simulink model "TDPBehaviourSim2"  (R2020b)
settings: Solver=FixedStepAuto  StartTime=0.0  StopTime=200  FixedStep=sampleTime  RelTol=1e-3  EnableMultiTasking=on
values from neighbouring files (symbols this model uses):
  angThresh = pi/16    (= 0.196349540849)    [GameParameters.m]
  attackerKickSpeed = 0.3    [GameParameters.m]
  AwayFormation1 = [9.5 4 pi ... (first row only)    [FormationPoses.m]    (also in GameParameters.m)
  ballAngleNoise = pi/24    (= 0.1308996939)    [GameParameters.m]
  ballThresh = playerRadius + 0.03    (= 0.11)    [GameParameters.m]
  ballVelNoise = 0.05    [GameParameters.m]
  distThresh = 0.1    [GameParameters.m]
  fieldCenter = [mean(fieldLimitsX) mean(fieldLimitsY)]    [GameParameters.m]
  fieldLimitsX = [1 10]    [GameParameters.m]
  fieldLimitsY = [1 7]    [GameParameters.m]
  goalPosts = [1  2.7 2 ... (first row only)    [GameParameters.m]
  HomeFormation1 = [1.5 4 0 ... (first row only)    [FormationPoses.m]    (also in GameParameters.m)
  maxSpeed = 0.1    [GameParameters.m]
  maxTurnSpeed = 0.05    [GameParameters.m]
  playerIdx = (0:8)    [GameParameters.m]
  playerRadius = 0.08    [GameParameters.m]
  sampleTime = 0.1    [GameParameters.m]
undefined symbols (not defined in the file or in its folder): DiscIntNeverNeededParam
libraries: mobileRoboticsLib x33, soccerRobotLib x16
(part 1 of 2)
settings Model: SimulationMode=accelerator  SnapshotBufferSize=20  Creator=2683935i  LastModifiedBy=2683935i
settings SolverCC: AutoInsertRateTranBlk=on
settings DataIOCC: SaveOutput=off  SaveTime=off
settings OptimizationCC: DefaultParameterBehavior=Inlined  InlineInvariantSignals=on  EnhancedBackFolding=on  PassReuseOutputArgsAs=Individual arguments  StateBitsets=on  DataBitsets=on  ZeroExternalMemoryAtStartup=off  ZeroInternalMemoryAtStartup=off  NoFixptDivByZeroProtection=on  LifeSpan=1  OptimizeBlockOrder=speed  DifferentSizesBufferReuse=on  EfficientTunableParamExpr=on
settings DebuggingCC: ParameterTunabilityLossMsg=error  UnderSpecifiedDimensionMsg=warning
settings HardwareCC: ProdBitPerPointer=32  ProdBitPerSizeT=32  ProdBitPerPtrDiffT=32  ProdLargestAtomicFloat=None  ProdIntDivRoundTo=Floor  ProdWordSize=32  ProdHWDeviceType=Generic->Custom
settings SFSimCC: MATLABDynamicMemAlloc=off
settings RTWCC: Description=Embedded Coder  SystemTargetFile=ert.tlc  TLCOptions=-p0  GenCodeOnly=on  TemplateMakefile=ert_default_tmf  GenerateReport=on  RTWVerbose=off  IncludeHyperlinkInReport=on  LaunchReport=on
settings CodeAppCC: ForceParamTrailComments=on  IgnoreCustomStorageClasses=off  OperatorAnnotations=on  SimulinkDataObjDesc=on  SFDataObjDesc=on  CustomSymbolStrGlobalVar=rt$N$M  CustomSymbolStrType=$N$M  CustomSymbolStrFcn=$N$M$F  CustomSymbolStrMacro=$N$M  InsertBlockDesc=on
settings ERTTargetCC: TargetLangStandard=C99 (ISO)  GenerateSampleERTMain=on  IncludeMdlTerminateFcn=off  SuppressErrorStatus=on  SupportAbsoluteTime=off  PurelyIntegerCode=on  SupportNonFinite=off  SupportComplex=off  InlinedParameterPlacement=NonHierarchical  RootIOFormat=Structure reference  ERTCustomFileTemplate=example_file_process.tlc

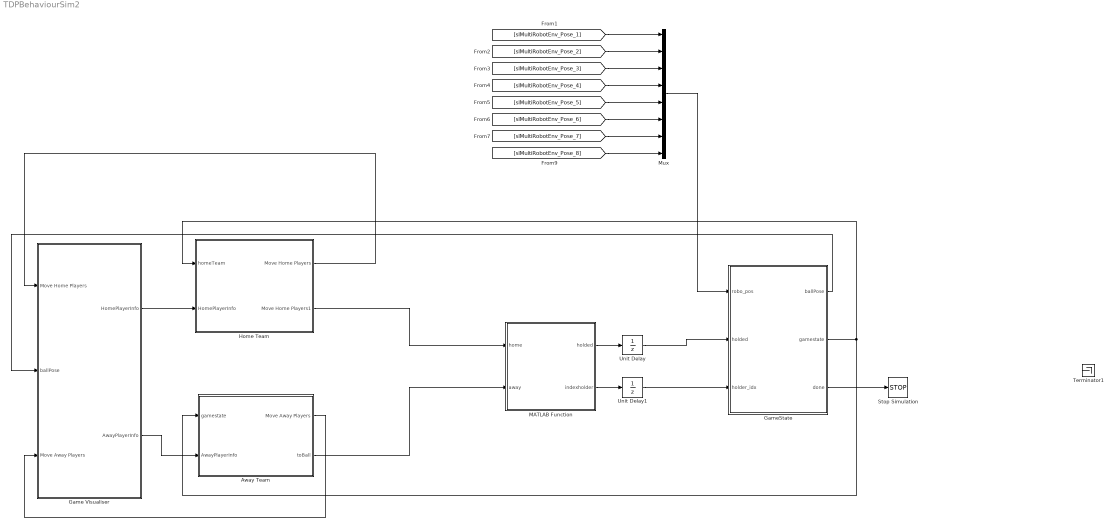
== system TDPBehaviourSim2 ==
  Away Team : Subsystem
  Game Visualiser : Subsystem
  GameState : Stateflow chart  TreatAsAtomicUnit=on
  Home Team : Subsystem
  MATLAB Function : MATLAB Function  TreatAsAtomicUnit=on
  Mux : Mux  Inputs=8
  Stop Simulation : Stop
  Terminator1 : Terminator
  Unit Delay : UnitDelay  SampleTime=-1  HasFrameUpgradeWarning=on
  Unit Delay1 : UnitDelay  SampleTime=-1  HasFrameUpgradeWarning=on
  wires:
  Home Team/1(Move Home Players) -> Game Visualiser/1(Move Home Players)
  Game Visualiser/1(HomePlayerInfo) -> Home Team/2(HomePlayerInfo)
  Game Visualiser/2(AwayPlayerInfo) -> Away Team/2(AwayPlayerInfo)
  [slMultiRobotEnv_Pose_4] -> Mux/4
  [slMultiRobotEnv_Pose_8] -> Mux/8
  [slMultiRobotEnv_Pose_1] -> Mux/1
  Mux/1 -> GameState/1(robo_pos)
  [slMultiRobotEnv_Pose_2] -> Mux/2
  [slMultiRobotEnv_Pose_3] -> Mux/3
  GameState/1(ballPose) -> Game Visualiser/2(ballPose)
  Home Team/2(Move Home Players1) -> MATLAB Function/1(home)
  GameState/3(done) -> Stop Simulation/1
  [slMultiRobotEnv_Pose_5] -> Mux/5
  [slMultiRobotEnv_Pose_6] -> Mux/6
  [slMultiRobotEnv_Pose_7] -> Mux/7
  GameState/2(gamestate) -> Away Team/1(gamestate), Home Team/1(homeTeam)
  MATLAB Function/2(indexholder) -> Unit Delay1/1
  Unit Delay1/1 -> GameState/3(holder_idx)
  MATLAB Function/1(holded) -> Unit Delay/1
  Unit Delay/1 -> GameState/2(holded)
  Away Team/2(toBall) -> MATLAB Function/2(away)
  Away Team/1(Move Away Players) -> Game Visualiser/3(Move Away Players)

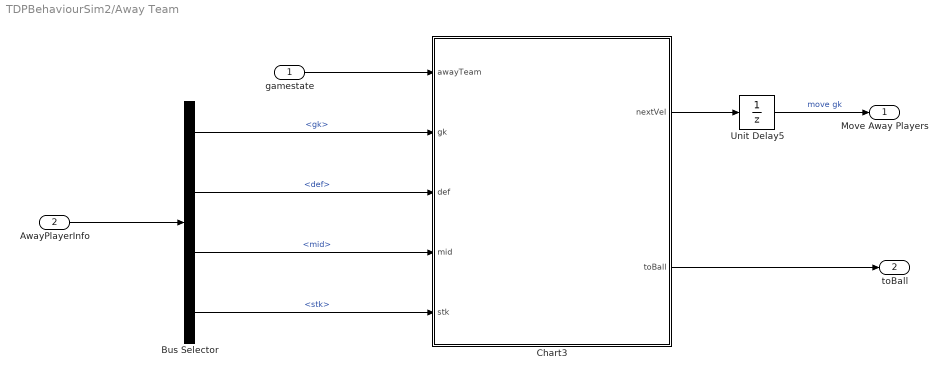
== system TDPBehaviourSim2/Away Team ==
  gamestate : Inport
  AwayPlayerInfo : Inport  Port=2
  Bus Selector : BusSelector  OutputSignals=gk,def,mid,stk
  Chart3 : Stateflow chart  TreatAsAtomicUnit=on
      settings: PortSchema="{\"entries\":[{\"content\":{\"sides\":[{\"content\":{\"connectorIds\":[\"In1\",\"In2\",\"In3\",\"In4\",\"In5\"]},\"type\":\"ConnectorPlacement.EquallySpacedRectSide\",\"uuid\":\"ebe0e1cb-6371-4bd3-ace0-cc5b71048631\"},{\"content\":{\"connectorIds\":[\"Out2\",\"Out1\"],\"side\":\"RIGHT\"},\"type\":\"ConnectorPlacement.EquallySpacedRectSide\",\"uuid\":\"57a2731b-5a64-47ed-8ccc-f0829cfb4352\"},{\"content\":{\"connectorIds\":[],\"side\":\"TOP\"},\"type\":\"ConnectorPlacement.EquallySpacedRectSide\",\"uuid\":\"36798d0f-f2da-4938-9b0d-f712c5a2717d\"},{\"content\":{\"connectorIds\":[],\"side\":\"HIDDEN\"},\"type\":\"ConnectorPlacement.EquallySpacedRectSide\",\"uuid\":\"e7d6e691-e5a0-4113-9f42-d5d110a4eaa7\"}]},\"type\":\"ConnectorPlacement.EquallySpacedConnector\",\"uuid\":\"d2e32adf-2fdb-404f-9614-4542aac92af5\"}],\"packageUris\":[\"http://schema.mathworks.com/mf0/Connector/R2020b\"],\"version\":\"1.0\"}"
  Unit Delay5 : UnitDelay  SampleTime=-1  HasFrameUpgradeWarning=on
  Move Away Players : Outport
  toBall : Outport  Port=2
  wires:
  Chart3/2(nextVel) -> Unit Delay5/1
  Unit Delay5/1 -> Move Away Players/1  "move gk"
  gamestate/1 -> Chart3/1(awayTeam)
  AwayPlayerInfo/1 -> Bus Selector/1
  Chart3/1(toBall) -> toBall/1
  Bus Selector/1 -> Chart3/2(gk)  "<gk>"
  Bus Selector/2 -> Chart3/3(def)  "<def>"
  Bus Selector/3 -> Chart3/4(mid)  "<mid>"
  Bus Selector/4 -> Chart3/5(stk)  "<stk>"

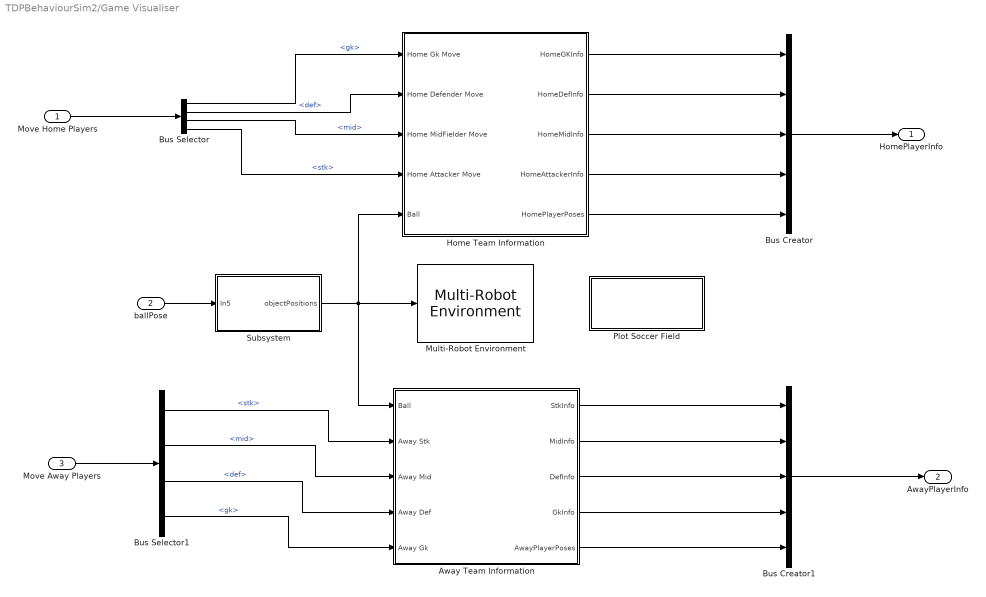
== system TDPBehaviourSim2/Game Visualiser ==
  Move Home Players : Inport
  ballPose : Inport  Port=2
  Move Away Players : Inport  Port=3
  Away Team Information : Subsystem
  Bus Creator : BusCreator  Inputs=5
  Bus Creator1 : BusCreator  Inputs=5
  Bus Selector : BusSelector  OutputSignals=gk,def,mid,stk
  Bus Selector1 : BusSelector  OutputSignals=stk,mid,def,gk
  Home Team Information : Subsystem
  Multi-Robot Environment : mobileRoboticsLib/Environments/Multi-Robot Environment  numRobots=numPlayers  mapName=map  showWaypoints=off  showObjects=on  objectColors=objColors  objectMarkers='o^^^^'  showRobotIds=on  plotSensorLines=off
      settings: SourceProductName=Mobile Robotics Simulation Toolbox
  Plot Soccer Field : MATLAB Function  TreatAsAtomicUnit=on
  Subsystem : Subsystem
  HomePlayerInfo : Outport
  AwayPlayerInfo : Outport  Port=2
  wires:
  Home Team Information/1(HomeGKInfo) -> Bus Creator/1
  Home Team Information/2(HomeDefInfo) -> Bus Creator/2
  Home Team Information/3(HomeMidInfo) -> Bus Creator/3
  Home Team Information/4(HomeAttackerInfo) -> Bus Creator/4
  Home Team Information/5(HomePlayerPoses) -> Bus Creator/5
  Away Team Information/1(StkInfo) -> Bus Creator1/1
  Away Team Information/2(MidInfo) -> Bus Creator1/2
  Away Team Information/3(DefInfo) -> Bus Creator1/3
  Away Team Information/4(GkInfo) -> Bus Creator1/4
  Away Team Information/5(AwayPlayerPoses) -> Bus Creator1/5
  Subsystem/1(objectPositions) -> Multi-Robot Environment/1, Away Team Information/1(Ball), Home Team Information/5(Ball)
  ballPose/1 -> Subsystem/1(In5)
  Move Away Players/1 -> Bus Selector1/1
  Bus Creator/1 -> HomePlayerInfo/1
  Bus Creator1/1 -> AwayPlayerInfo/1
  Move Home Players/1 -> Bus Selector/1
  Bus Selector/1 -> Home Team Information/1(Home Gk Move)  "<gk>"
  Bus Selector/2 -> Home Team Information/2(Home Defender Move)  "<def>"
  Bus Selector/3 -> Home Team Information/3(Home MidFielder Move)  "<mid>"
  Bus Selector/4 -> Home Team Information/4(Home Attacker Move)  "<stk>"
  Bus Selector1/1 -> Away Team Information/2(Away Stk)  "<stk>"
  Bus Selector1/2 -> Away Team Information/3(Away Mid)  "<mid>"
  Bus Selector1/3 -> Away Team Information/4(Away Def)  "<def>"
  Bus Selector1/4 -> Away Team Information/5("Away Gk ")  "<gk>"

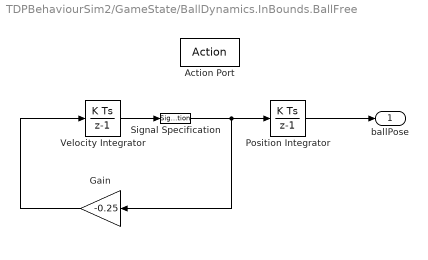
== system TDPBehaviourSim2/GameState/BallDynamics.InBounds.BallFree ==
  Action Port : ActionPort
      settings: CopyFcn=Stateflow.SLINSF.SimulinkMan.removeBlockPreDeleteFcn  PreDeleteFcn=Stateflow.SLINSF.SimulinkMan.unsafePredeleteFcn
  Gain : Gain  Gain=-0.25
  Position Integrator : DiscreteIntegrator  InitialCondition=fieldCenter  SampleTime=-1  StateName=ballPos  ICPrevOutput=DiscIntNeverNeededParam  ICPrevScaledInput=DiscIntNeverNeededParam
  Signal Specification : SignalSpecification  Dimensions=[1 2]
  Velocity Integrator : DiscreteIntegrator  InitialCondition=[0 0]  SampleTime=-1  StateName=ballVel  ICPrevOutput=DiscIntNeverNeededParam  ICPrevScaledInput=DiscIntNeverNeededParam
  ballPose : Outport  VectorParamsAs1DForOutWhenUnconnected=off
  wires:
  Gain/1 -> Velocity Integrator/1
  Velocity Integrator/1 -> Signal Specification/1
  Position Integrator/1 -> ballPose/1
  Signal Specification/1 -> Position Integrator/1, Gain/1

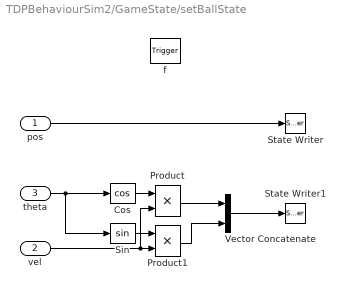
== system TDPBehaviourSim2/GameState/setBallState ==
  pos : Inport  OutDataTypeStr=double  PortDimensions=[1 2]
  vel : Inport  Port=2  OutDataTypeStr=double  PortDimensions=1
  theta : Inport  Port=3  OutDataTypeStr=double  PortDimensions=1
  f : TriggerPort  TriggerType=function-call  VariantControl=(inherit)
      settings: CopyFcn=Stateflow.SLINSF.SimulinkMan.removeBlockPreDeleteFcn  PreDeleteFcn=Stateflow.SLINSF.SimulinkMan.unsafePredeleteFcn
  Cos : Trigonometry  Operator=cos
  Product : Product
  Product1 : Product
  Sin : Trigonometry
  State Writer : StateWriter  StateOwnerBlock=../../BallDynamics.InBounds.BallFree/Position Integrator  StateName=ballPos
  State Writer1 : StateWriter  StateOwnerBlock=../../BallDynamics.InBounds.BallFree/Velocity Integrator  StateName=ballVel
  Vector Concatenate : Concatenate  Mode=Multidimensional array  ConcatenateDimension=2
  wires:
  Vector Concatenate/1 -> State Writer1/1
  Product1/1 -> Vector Concatenate/2
  Product/1 -> Vector Concatenate/1
  theta/1 -> Cos/1, Sin/1
  Sin/1 -> Product1/1
  vel/1 -> Product1/2, Product/2
  Cos/1 -> Product/1
  pos/1 -> State Writer/1

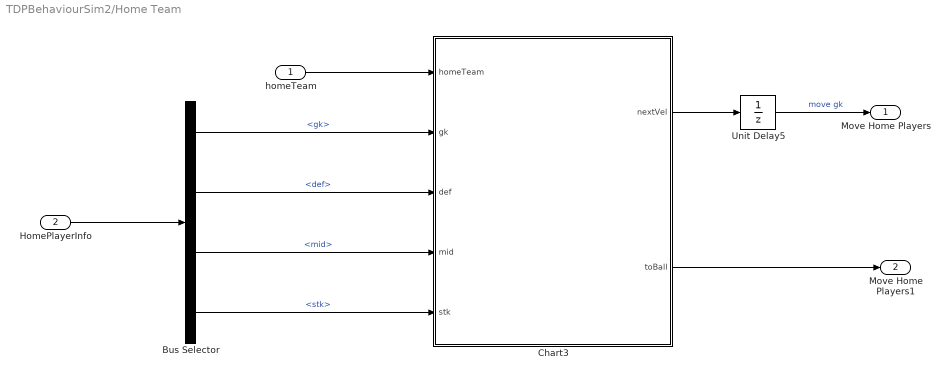
== system TDPBehaviourSim2/Home Team ==
  homeTeam : Inport
  HomePlayerInfo : Inport  Port=2
  Bus Selector : BusSelector  OutputSignals=gk,def,mid,stk
  Chart3 : Stateflow chart  TreatAsAtomicUnit=on
      settings: PortSchema="{\"entries\":[{\"content\":{\"sides\":[{\"content\":{\"connectorIds\":[\"In1\",\"In2\",\"In3\",\"In4\",\"In5\"]},\"type\":\"ConnectorPlacement.EquallySpacedRectSide\",\"uuid\":\"ebe0e1cb-6371-4bd3-ace0-cc5b71048631\"},{\"content\":{\"connectorIds\":[\"Out2\",\"Out1\"],\"side\":\"RIGHT\"},\"type\":\"ConnectorPlacement.EquallySpacedRectSide\",\"uuid\":\"57a2731b-5a64-47ed-8ccc-f0829cfb4352\"},{\"content\":{\"connectorIds\":[],\"side\":\"TOP\"},\"type\":\"ConnectorPlacement.EquallySpacedRectSide\",\"uuid\":\"36798d0f-f2da-4938-9b0d-f712c5a2717d\"},{\"content\":{\"connectorIds\":[],\"side\":\"HIDDEN\"},\"type\":\"ConnectorPlacement.EquallySpacedRectSide\",\"uuid\":\"e7d6e691-e5a0-4113-9f42-d5d110a4eaa7\"}]},\"type\":\"ConnectorPlacement.EquallySpacedConnector\",\"uuid\":\"d2e32adf-2fdb-404f-9614-4542aac92af5\"}],\"packageUris\":[\"http://schema.mathworks.com/mf0/Connector/R2020b\"],\"version\":\"1.0\"}"
  Unit Delay5 : UnitDelay  SampleTime=-1  HasFrameUpgradeWarning=on
  Move Home Players : Outport
  Move Home Players1 : Outport  Port=2
  wires:
  HomePlayerInfo/1 -> Bus Selector/1
  Bus Selector/2 -> Chart3/3(def)  "<def>"
  Bus Selector/3 -> Chart3/4(mid)  "<mid>"
  Bus Selector/4 -> Chart3/5(stk)  "<stk>"
  Bus Selector/1 -> Chart3/2(gk)  "<gk>"
  Chart3/1(toBall) -> Move Home Players1/1
  Chart3/2(nextVel) -> Unit Delay5/1
  Unit Delay5/1 -> Move Home Players/1  "move gk"
  homeTeam/1 -> Chart3/1(homeTeam)

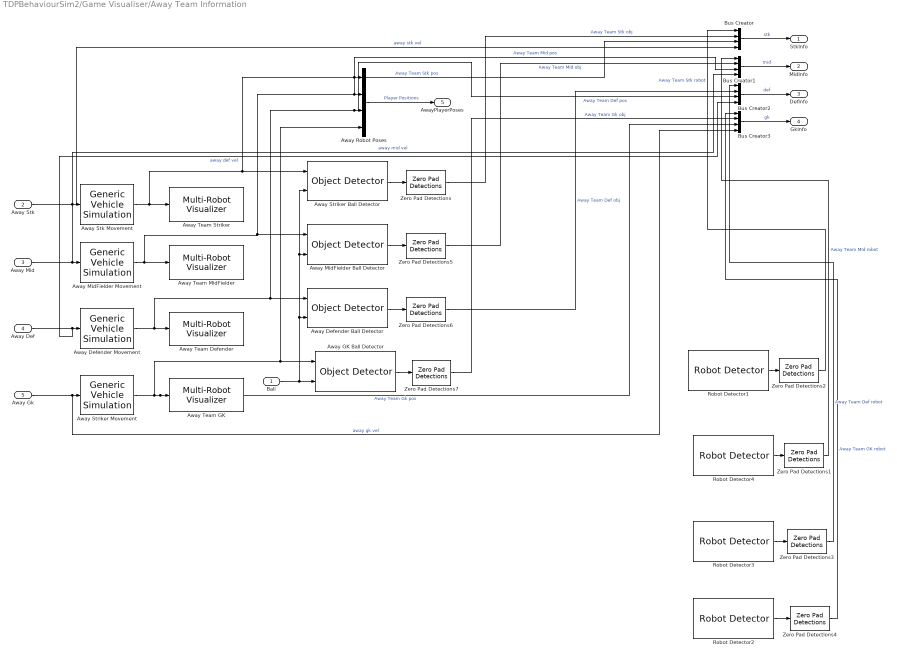
== system TDPBehaviourSim2/Game Visualiser/Away Team Information ==
  Ball : Inport
  Away Stk : Inport  Port=2
  Away Mid : Inport  Port=3
  Away Def : Inport  Port=4
  "Away Gk " : Inport  Port=5
  Away Defender Ball Detector : mobileRoboticsLib/Environments/Object Detector  mapName=map  sensorOffset=objDetectorOffset  sensorAngle=objDetectorAngle  fieldOfView=objDetectorFOV  maxRange=objDetectorRange  maxDetections=objDetectorMaxHits  sampleTime=sampleTime
      settings: SourceProductName=Mobile Robotics Simulation Toolbox
  Away Defender Movement : mobileRoboticsLib/Utilities/Generic Vehicle Simulation  initX=AwayFormation1(2,1)  initY=AwayFormation1(2,2)  initAngle=AwayFormation1(2,3)  Ts=sampleTime
      settings: SourceProductName=Mobile Robotics Simulation Toolbox
  Away GK Ball Detector : mobileRoboticsLib/Environments/Object Detector  mapName=map  sensorOffset=objDetectorOffset  sensorAngle=objDetectorAngle  fieldOfView=objDetectorFOV  maxRange=objDetectorRange  maxDetections=objDetectorMaxHits  sampleTime=sampleTime
      settings: SourceProductName=Mobile Robotics Simulation Toolbox
  Away MidFielder Ball Detector : mobileRoboticsLib/Environments/Object Detector  mapName=map  sensorOffset=objDetectorOffset  sensorAngle=objDetectorAngle  fieldOfView=objDetectorFOV  maxRange=objDetectorRange  maxDetections=objDetectorMaxHits  sampleTime=sampleTime
      settings: SourceProductName=Mobile Robotics Simulation Toolbox
  Away MidFielder Movement : mobileRoboticsLib/Utilities/Generic Vehicle Simulation  initX=AwayFormation1(3,1)  initY=AwayFormation1(3,2)  initAngle=AwayFormation1(3,3)  Ts=sampleTime
      settings: SourceProductName=Mobile Robotics Simulation Toolbox
  Away Robot Poses : BusCreator  Inputs=4
  Away Stk Movement : mobileRoboticsLib/Utilities/Generic Vehicle Simulation  initX=AwayFormation1(4,1)  initY=AwayFormation1(4,2)  initAngle=AwayFormation1(4,3)  Ts=sampleTime
      settings: SourceProductName=Mobile Robotics Simulation Toolbox
  Away Striker Ball Detector : mobileRoboticsLib/Environments/Object Detector  mapName=map  sensorOffset=objDetectorOffset  sensorAngle=objDetectorAngle  fieldOfView=objDetectorFOV  maxRange=objDetectorRange  maxDetections=objDetectorMaxHits  sampleTime=sampleTime
      settings: SourceProductName=Mobile Robotics Simulation Toolbox
  Away Striker Movement : mobileRoboticsLib/Utilities/Generic Vehicle Simulation  initX=AwayFormation1(1,1)  initY=AwayFormation1(1,2)  initAngle=AwayFormation1(1,3)  Ts=sampleTime
      settings: SourceProductName=Mobile Robotics Simulation Toolbox
  Away Team Defender : mobileRoboticsLib/Environments/Multi-Robot Visualizer  idx=7  radius=playerRadius  robotColor=awayTeamColor  showTraj=on  hasLidar=off  sensorOffset=[0,0]  scanAngles=[-pi/4 0 pi/4]  maxNumScans=0  hasObjDetector=on  objDetectorOffset=objDetectorOffset  objDetectorAngle=objDetectorAngle  objDetectorFOV=objDetectorFOV  objDetectorMaxRange=objDetectorRange  hasRobotDetector=on  robotDetectorOffset=robotDetectorOffset  robotDetectorAngle=robotDetectorAngle  robotDetectorFOV=robotDetectorFOV  robotDetectorMaxRange=robotDetectorMaxHits  robotDetectorNumDetections=0
      settings: SourceProductName=Mobile Robotics Simulation Toolbox
  Away Team GK : mobileRoboticsLib/Environments/Multi-Robot Visualizer  idx=8  radius=playerRadius  robotColor=awayGKColor  showTraj=on  hasLidar=off  sensorOffset=[0,0]  scanAngles=[-pi/4 0 pi/4]  maxNumScans=0  hasObjDetector=on  objDetectorOffset=objDetectorOffset  objDetectorAngle=objDetectorAngle  objDetectorFOV=objDetectorFOV  objDetectorMaxRange=objDetectorRange  hasRobotDetector=on  robotDetectorOffset=robotDetectorOffset  robotDetectorAngle=robotDetectorAngle  robotDetectorFOV=robotDetectorFOV  robotDetectorMaxRange=robotDetectorMaxHits  robotDetectorNumDetections=0
      settings: SourceProductName=Mobile Robotics Simulation Toolbox
  Away Team MidFielder : mobileRoboticsLib/Environments/Multi-Robot Visualizer  idx=6  radius=playerRadius  robotColor=awayTeamColor  showTraj=on  hasLidar=off  sensorOffset=[0,0]  scanAngles=[-pi/4 0 pi/4]  maxNumScans=0  hasObjDetector=on  objDetectorOffset=objDetectorOffset  objDetectorAngle=objDetectorAngle  objDetectorFOV=objDetectorFOV  objDetectorMaxRange=objDetectorRange  hasRobotDetector=on  robotDetectorOffset=robotDetectorOffset  robotDetectorAngle=robotDetectorAngle  robotDetectorFOV=robotDetectorFOV  robotDetectorMaxRange=robotDetectorMaxHits  robotDetectorNumDetections=0
      settings: SourceProductName=Mobile Robotics Simulation Toolbox
  Away Team Striker : mobileRoboticsLib/Environments/Multi-Robot Visualizer  idx=5  radius=playerRadius  robotColor=awayTeamColor  showTraj=on  hasLidar=off  sensorOffset=[0,0]  scanAngles=[-pi/4 0 pi/4]  maxNumScans=0  hasObjDetector=on  objDetectorOffset=objDetectorOffset  objDetectorAngle=objDetectorAngle  objDetectorFOV=objDetectorFOV  objDetectorMaxRange=objDetectorRange  hasRobotDetector=on  robotDetectorOffset=robotDetectorOffset  robotDetectorAngle=robotDetectorAngle  robotDetectorFOV=robotDetectorFOV  robotDetectorMaxRange=robotDetectorMaxHits  robotDetectorNumDetections=0
      settings: SourceProductName=Mobile Robotics Simulation Toolbox
  Bus Creator{,1..3} (4 alike) : BusCreator  Inputs=4  OutDataTypeStr=Bus: PlayerStateBus
      settings: InheritFromInputs=off
  Robot Detector1 : mobileRoboticsLib/Environments/Robot Detector  mapName=map  robotIdx=5  sensorOffset=robotDetectorOffset  sensorAngle=robotDetectorAngle  sensorFOV=robotDetectorFOV  maxRange=robotDetectorRange  maxDetections=robotDetectorMaxHits  sampleTime=sampleTime
      settings: SourceProductName=Mobile Robotics Simulation Toolbox
  Robot Detector2 : mobileRoboticsLib/Environments/Robot Detector  mapName=map  robotIdx=8  sensorOffset=robotDetectorOffset  sensorAngle=robotDetectorAngle  sensorFOV=robotDetectorFOV  maxRange=robotDetectorRange  maxDetections=robotDetectorMaxHits  sampleTime=sampleTime
      settings: SourceProductName=Mobile Robotics Simulation Toolbox
  Robot Detector3 : mobileRoboticsLib/Environments/Robot Detector  mapName=map  robotIdx=7  sensorOffset=robotDetectorOffset  sensorAngle=robotDetectorAngle  sensorFOV=robotDetectorFOV  maxRange=robotDetectorRange  maxDetections=robotDetectorMaxHits  sampleTime=sampleTime
      settings: SourceProductName=Mobile Robotics Simulation Toolbox
  Robot Detector4 : mobileRoboticsLib/Environments/Robot Detector  mapName=map  robotIdx=6  sensorOffset=robotDetectorOffset  sensorAngle=robotDetectorAngle  sensorFOV=robotDetectorFOV  maxRange=robotDetectorRange  maxDetections=robotDetectorMaxHits  sampleTime=sampleTime
      settings: SourceProductName=Mobile Robotics Simulation Toolbox
  Zero Pad Detections{,5..7} (4 alike) : soccerRobotLib/Soccer Robot Simulator/Zero Pad Detections  maxHits=objDetectorMaxHits
  Zero Pad Detections{1..4} (4 alike) : soccerRobotLib/Soccer Robot Simulator/Zero Pad Detections  maxHits=robotDetectorMaxHits
  StkInfo : Outport
  MidInfo : Outport  Port=2
  DefInfo : Outport  Port=3
  GkInfo : Outport  Port=4
  AwayPlayerPoses : Outport  Port=5
  wires:
  "Away Gk "/1 -> Bus Creator3/4, Away Striker Movement/1  "away gk vel"
  Away Def/1 -> Bus Creator2/4, Away Defender Movement/1  "away def vel"
  Ball/1 -> Away Defender Ball Detector/2, Away Striker Ball Detector/2, Away MidFielder Ball Detector/2, Away GK Ball Detector/2
  Away Striker Ball Detector/1 -> Zero Pad Detections/1
  Away Defender Ball Detector/1 -> Zero Pad Detections6/1
  Away MidFielder Ball Detector/1 -> Zero Pad Detections5/1
  Away GK Ball Detector/1 -> Zero Pad Detections7/1
  Zero Pad Detections/1 -> Bus Creator/2  "Away Team Stk obj"
  Zero Pad Detections5/1 -> Bus Creator1/2  "Away Team MId obj"
  Zero Pad Detections6/1 -> Bus Creator2/2  "Away Team Def obj"
  Zero Pad Detections7/1 -> Bus Creator3/2  "Away Team Gk obj"
  Away Striker Movement/1 -> Bus Creator3/3, Away Team GK/1, Away Robot Poses/4, Away GK Ball Detector/1  "Away Team Gk pos"
  Away MidFielder Movement/1 -> Away Team MidFielder/1, Away MidFielder Ball Detector/1, Bus Creator1/3, Away Robot Poses/2  "Away Team Mid pos"
  Away Stk Movement/1 -> Bus Creator/3, Away Robot Poses/1, Away Striker Ball Detector/1, Away Team Striker/1  "Away Team Stk pos"
  Away Defender Movement/1 -> Away Defender Ball Detector/1, Bus Creator2/3, Away Robot Poses/3, Away Team Defender/1  "Away Team Def pos"
  Zero Pad Detections1/1 -> Bus Creator1/1  "Away Team MId robot"
  Zero Pad Detections3/1 -> Bus Creator2/1  "Away Team Def robot"
  Robot Detector1/1 -> Zero Pad Detections2/1
  Robot Detector4/1 -> Zero Pad Detections1/1
  Robot Detector3/1 -> Zero Pad Detections3/1
  Robot Detector2/1 -> Zero Pad Detections4/1
  Zero Pad Detections4/1 -> Bus Creator3/1  "Away Team GK robot"
  Zero Pad Detections2/1 -> Bus Creator/1  "Away Team Stk robot"
  Away Stk/1 -> Bus Creator/4, Away Stk Movement/1  "away stk vel"
  Away Mid/1 -> Bus Creator1/4, Away MidFielder Movement/1  "away mid vel"
  Bus Creator/1 -> StkInfo/1  "stk"
  Bus Creator1/1 -> MidInfo/1  "mid"
  Bus Creator2/1 -> DefInfo/1  "def"
  Bus Creator3/1 -> GkInfo/1  "gk"
  Away Robot Poses/1 -> AwayPlayerPoses/1  "Player Positions"

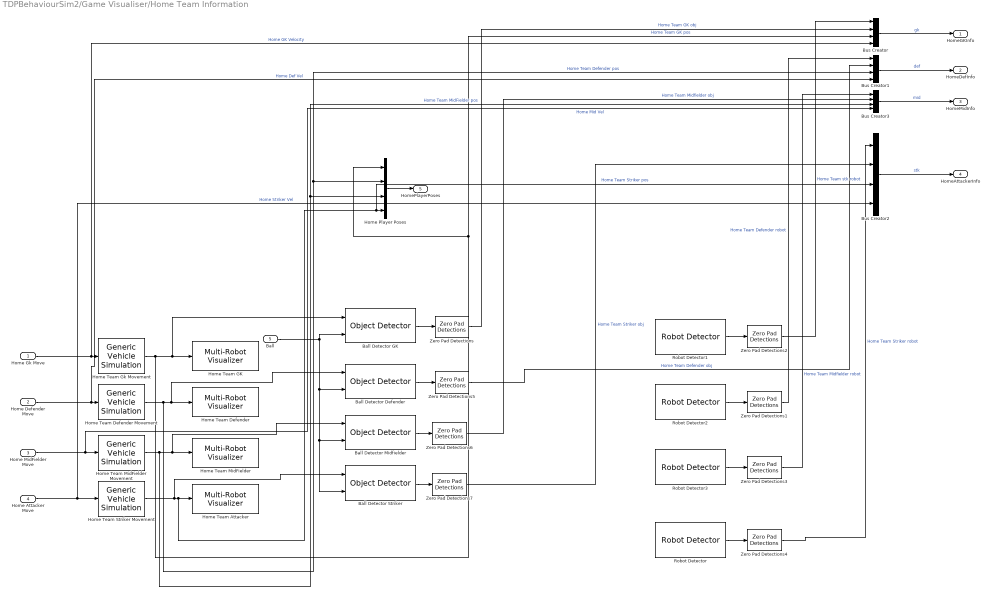
== system TDPBehaviourSim2/Game Visualiser/Home Team Information ==
  Home Gk Move : Inport
  Home Defender Move : Inport  Port=2
  Home MidFielder Move : Inport  Port=3
  Home Attacker Move : Inport  Port=4
  Ball : Inport  Port=5
  Ball Detector Defender : mobileRoboticsLib/Environments/Object Detector  mapName=map  sensorOffset=objDetectorOffset  sensorAngle=objDetectorAngle  fieldOfView=objDetectorFOV  maxRange=objDetectorRange  maxDetections=objDetectorMaxHits  sampleTime=sampleTime
      settings: SourceProductName=Mobile Robotics Simulation Toolbox
  Ball Detector GK : mobileRoboticsLib/Environments/Object Detector  mapName=map  sensorOffset=objDetectorOffset  sensorAngle=objDetectorAngle  fieldOfView=objDetectorFOV  maxRange=objDetectorRange  maxDetections=objDetectorMaxHits  sampleTime=sampleTime
      settings: SourceProductName=Mobile Robotics Simulation Toolbox
  Ball Detector Midfielder : mobileRoboticsLib/Environments/Object Detector  mapName=map  sensorOffset=objDetectorOffset  sensorAngle=objDetectorAngle  fieldOfView=objDetectorFOV  maxRange=objDetectorRange  maxDetections=objDetectorMaxHits  sampleTime=sampleTime
      settings: SourceProductName=Mobile Robotics Simulation Toolbox
  Ball Detector Striker : mobileRoboticsLib/Environments/Object Detector  mapName=map  sensorOffset=objDetectorOffset  sensorAngle=objDetectorAngle  fieldOfView=objDetectorFOV  maxRange=objDetectorRange  maxDetections=objDetectorMaxHits  sampleTime=sampleTime
      settings: SourceProductName=Mobile Robotics Simulation Toolbox
  Bus Creator{,1..3} (4 alike) : BusCreator  Inputs=4  OutDataTypeStr=Bus: PlayerStateBus
      Bus Creator settings: InheritFromInputs=off
  Home Player Poses : BusCreator  Inputs=4
  Home Team Attacker : mobileRoboticsLib/Environments/Multi-Robot Visualizer  idx=4  radius=playerRadius  robotColor=homeTeamColor  showTraj=on  hasLidar=off  sensorOffset=[0,0]  scanAngles=[-pi/4 0 pi/4]  maxNumScans=0  hasObjDetector=on  objDetectorOffset=objDetectorOffset  objDetectorAngle=objDetectorAngle  objDetectorFOV=objDetectorFOV  objDetectorMaxRange=objDetectorMaxHits  hasRobotDetector=on  robotDetectorOffset=robotDetectorOffset  robotDetectorAngle=robotDetectorAngle  robotDetectorFOV=robotDetectorFOV  robotDetectorMaxRange=robotDetectorRange  robotDetectorNumDetections=0
      settings: SourceProductName=Mobile Robotics Simulation Toolbox
  Home Team Defender : mobileRoboticsLib/Environments/Multi-Robot Visualizer  idx=2  radius=playerRadius  robotColor=homeTeamColor  showTraj=on  hasLidar=off  sensorOffset=[0,0]  scanAngles=[-pi/4 0 pi/4]  maxNumScans=0  hasObjDetector=on  objDetectorOffset=objDetectorOffset  objDetectorAngle=objDetectorAngle  objDetectorFOV=objDetectorFOV  objDetectorMaxRange=objDetectorMaxHits  hasRobotDetector=off  robotDetectorOffset=[0,0]  robotDetectorAngle=0  robotDetectorFOV=pi/3  robotDetectorMaxRange=5  robotDetectorNumDetections=0
      settings: SourceProductName=Mobile Robotics Simulation Toolbox
  Home Team Defender Movement : mobileRoboticsLib/Utilities/Generic Vehicle Simulation  initX=HomeFormation1(2,1)  initY=HomeFormation1(2,2)  initAngle=HomeFormation1(2,3)  Ts=sampleTime
      settings: SourceProductName=Mobile Robotics Simulation Toolbox
  Home Team GK : mobileRoboticsLib/Environments/Multi-Robot Visualizer  idx=1  radius=playerRadius  robotColor=homeGKColor  showTraj=on  hasLidar=off  sensorOffset=[0,0]  scanAngles=[-pi/4 0 pi/4]  maxNumScans=0  hasObjDetector=on  objDetectorOffset=objDetectorOffset  objDetectorAngle=objDetectorAngle  objDetectorFOV=objDetectorFOV  objDetectorMaxRange=objDetectorRange  hasRobotDetector=on  robotDetectorOffset=robotDetectorOffset  robotDetectorAngle=robotDetectorAngle  robotDetectorFOV=robotDetectorFOV  robotDetectorMaxRange=robotDetectorRange  robotDetectorNumDetections=0
      settings: SourceProductName=Mobile Robotics Simulation Toolbox
  Home Team Gk Movement : mobileRoboticsLib/Utilities/Generic Vehicle Simulation  initX=HomeFormation1(1,1)  initY=HomeFormation1(1,2)  initAngle=HomeFormation1(1,3)  Ts=sampleTime
      settings: SourceProductName=Mobile Robotics Simulation Toolbox
  Home Team MidFielder : mobileRoboticsLib/Environments/Multi-Robot Visualizer  idx=3  radius=playerRadius  robotColor=homeTeamColor  showTraj=on  hasLidar=off  sensorOffset=[0,0]  scanAngles=[-pi/4 0 pi/4]  maxNumScans=0  hasObjDetector=off  objDetectorOffset=[0,0]  objDetectorAngle=0  objDetectorFOV=pi/3  objDetectorMaxRange=5  hasRobotDetector=off  robotDetectorOffset=[0,0]  robotDetectorAngle=0  robotDetectorFOV=pi/3  robotDetectorMaxRange=5  robotDetectorNumDetections=0
      settings: SourceProductName=Mobile Robotics Simulation Toolbox
  Home Team MidFielder Movement : mobileRoboticsLib/Utilities/Generic Vehicle Simulation  initX=HomeFormation1(3,1)  initY=HomeFormation1(3,2)  initAngle=HomeFormation1(3,3)  Ts=sampleTime
      settings: SourceProductName=Mobile Robotics Simulation Toolbox
  Home Team Striker Movement : mobileRoboticsLib/Utilities/Generic Vehicle Simulation  initX=HomeFormation1(4,1)  initY=HomeFormation1(4,2)  initAngle=HomeFormation1(4,3)  Ts=sampleTime
      settings: SourceProductName=Mobile Robotics Simulation Toolbox
  Robot Detector : mobileRoboticsLib/Environments/Robot Detector  mapName=map  robotIdx=4  sensorOffset=robotDetectorOffset  sensorAngle=robotDetectorAngle  sensorFOV=robotDetectorFOV  maxRange=robotDetectorRange  maxDetections=robotDetectorMaxHits  sampleTime=sampleTime
      settings: SourceProductName=Mobile Robotics Simulation Toolbox
  Robot Detector1 : mobileRoboticsLib/Environments/Robot Detector  mapName=map  robotIdx=1  sensorOffset=robotDetectorOffset  sensorAngle=robotDetectorAngle  sensorFOV=robotDetectorFOV  maxRange=robotDetectorRange  maxDetections=robotDetectorMaxHits  sampleTime=sampleTime
      settings: SourceProductName=Mobile Robotics Simulation Toolbox
  Robot Detector2 : mobileRoboticsLib/Environments/Robot Detector  mapName=map  robotIdx=2  sensorOffset=robotDetectorOffset  sensorAngle=robotDetectorAngle  sensorFOV=robotDetectorFOV  maxRange=robotDetectorRange  maxDetections=robotDetectorMaxHits  sampleTime=sampleTime
      settings: SourceProductName=Mobile Robotics Simulation Toolbox
  Robot Detector3 : mobileRoboticsLib/Environments/Robot Detector  mapName=map  robotIdx=3  sensorOffset=robotDetectorOffset  sensorAngle=robotDetectorAngle  sensorFOV=robotDetectorFOV  maxRange=robotDetectorRange  maxDetections=robotDetectorMaxHits  sampleTime=sampleTime
      settings: SourceProductName=Mobile Robotics Simulation Toolbox
  Zero Pad Detections{,5..7} (4 alike) : soccerRobotLib/Soccer Robot Simulator/Zero Pad Detections  maxHits=objDetectorMaxHits
  Zero Pad Detections{1..4} (4 alike) : soccerRobotLib/Soccer Robot Simulator/Zero Pad Detections  maxHits=robotDetectorMaxHits
  HomeGKInfo : Outport
  HomeDefInfo : Outport  Port=2
  HomeMidInfo : Outport  Port=3
  HomeAttackerInfo : Outport  Port=4
  HomePlayerPoses : Outport  Port=5
  wires:
  Home Gk Move/1 -> Bus Creator/4, Home Team Gk Movement/1  "Home GK Velocity"
  Home Team Striker Movement/1 -> Bus Creator2/3, Home Player Poses/4, Home Team Attacker/1, Ball Detector Striker/1  "Home Team Striker pos"
  Home Attacker Move/1 -> Bus Creator2/4, Home Team Striker Movement/1  "Home Striker Vel"
  Home Defender Move/1 -> Bus Creator1/4, Home Team Defender Movement/1  "Home Def Vel"
  Home Team Gk Movement/1 -> Ball Detector GK/1, Home Team GK/1, Bus Creator/3, Home Player Poses/1  "Home Team GK pos"
  Home Team Defender Movement/1 -> Bus Creator1/3, Home Player Poses/2, Ball Detector Defender/1, Home Team Defender/1  "Home Team Defender pos"
  Home Team MidFielder Movement/1 -> Bus Creator3/3, Home Player Poses/3, Ball Detector Midfielder/1, Home Team MidFielder/1  "Home Team MidFielder pos"
  Home MidFielder Move/1 -> Bus Creator3/4, Home Team MidFielder Movement/1  "Home Mid Vel"
  Ball/1 -> Ball Detector GK/2, Ball Detector Striker/2, Ball Detector Midfielder/2, Ball Detector Defender/2
  Ball Detector GK/1 -> Zero Pad Detections/1
  Ball Detector Midfielder/1 -> Zero Pad Detections6/1
  Ball Detector Defender/1 -> Zero Pad Detections5/1
  Ball Detector Striker/1 -> Zero Pad Detections7/1
  Robot Detector1/1 -> Zero Pad Detections2/1
  Robot Detector3/1 -> Zero Pad Detections3/1
  Robot Detector/1 -> Zero Pad Detections4/1
  Zero Pad Detections/1 -> Bus Creator/2  "Home Team GK obj"
  Zero Pad Detections2/1 -> Bus Creator/1  "Home Team stk robot"
  Zero Pad Detections1/1 -> Bus Creator1/1  "Home Team Defender robot"
  Robot Detector2/1 -> Zero Pad Detections1/1
  Zero Pad Detections3/1 -> Bus Creator3/1  "Home Team Midfielder robot"
  Zero Pad Detections4/1 -> Bus Creator2/1  "Home Team Striker robot"
  Zero Pad Detections5/1 -> Bus Creator1/2  "Home Team Defender obj"
  Zero Pad Detections6/1 -> Bus Creator3/2  "Home Team Midfielder obj"
  Zero Pad Detections7/1 -> Bus Creator2/2  "Home Team Striker obj"
  Home Player Poses/1 -> HomePlayerPoses/1
  Bus Creator/1 -> HomeGKInfo/1  "gk"
  Bus Creator1/1 -> HomeDefInfo/1  "def"
  Bus Creator3/1 -> HomeMidInfo/1  "mid"
  Bus Creator2/1 -> HomeAttackerInfo/1  "stk"

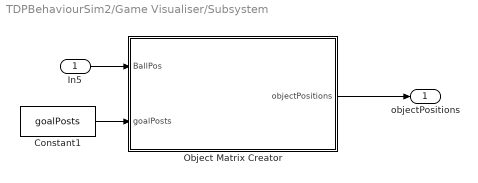
== system TDPBehaviourSim2/Game Visualiser/Subsystem ==
  In5 : Inport
  Constant1 : Constant  Value=goalPosts
  Object Matrix Creator : MATLAB Function  TreatAsAtomicUnit=on
  objectPositions : Outport
  wires:
  Constant1/1 -> Object Matrix Creator/2(goalPosts)
  In5/1 -> Object Matrix Creator/1(BallPos)
  Object Matrix Creator/1(objectPositions) -> objectPositions/1

== stateflow chart TDPBehaviourSim2/Away Team/Chart3 ==
  state BallInteraction [parallel]
    en,du:
    toBall = [gkObjSeen,gkObjDist,gkObjAng;
    defObjSeen,defObjDist,defObjAng;
    midObjSeen,midObjDist,midObjAng;
    stkObjSeen,stkObjDist,stkObjAng]
    settings: executionOrder=2
  state MoveTeam [parallel]
    en,du:
    settings: executionOrder=1
    state Attack
      en,du:
      state GoalKeeper [parallel]
        en,du:
        [gkObjSeen,gkObjDist,gkObjAng]=detectObj(gk.objectDetections,1)
        settings: executionOrder=1
      state Defender [parallel]
        en,du:
        [defObjSeen,defObjDist,defObjAng]=detectObj(def.objectDetections,1);
        settings: executionOrder=2
      state MidFielder [parallel]
        en,du:
        [midObjSeen,midObjDist,midObjAng]=detectObj(mid.objectDetections,1);
        settings: executionOrder=3
      state Striker [parallel]
        en,du:
        [stkObjSeen,stkObjDist,stkObjAng]=detectObj(stk.objectDetections,1)
        settings: executionOrder=4
        state InPossession
          en,du:
          nextVel.stk = goToPose([8,4,pi],stk.position);
        state TeammateInPossession
          en,du:
        (default) -> (junction 231)
        (junction 231) -> InPossession [order 1] : [awayTeam.possession(1)==1 &&...
            | awayTeam.possession(2)==playerIdx(5)]
        (junction 231) -> (junction 236) [order 2]
        InPossession -> TeammateInPossession : [awayTeam.possession(1)==1 &&...
            | awayTeam.possession(2)~=playerIdx(5)]
        TeammateInPossession -> InPossession : [awayTeam.possession(1)==1 &&...
            | awayTeam.possession(2)==playerIdx(5)]
        (junction 236) -> TeammateInPossession
    state Defend
      en,du:
      state GoalKeeper [parallel]
        en,du:
        [gkObjSeen,gkObjDist,gkObjAng]=detectObj(gk.objectDetections,1)
        settings: executionOrder=3
      state Defender [parallel]
        en,du:
        [defObjSeen,defObjDist,defObjAng]=detectObj(def.objectDetections,1);
        settings: executionOrder=4
      state MidFielder [parallel]
        en,du:
        [midObjSeen,midObjDist,midObjAng]=detectObj(mid.objectDetections,1);
        settings: executionOrder=1
      state Striker [parallel]
        en,du:
        [stkObjSeen,stkObjDist,stkObjAng]=detectObj(stk.objectDetections,1)
        settings: executionOrder=2
    state CaptureBall
      en,du:
      state GoalKeeper [parallel]
        en,du:
        [gkObjSeen,gkObjDist,gkObjAng]=detectObj(gk.objectDetections,1)
        settings: executionOrder=3
      state Defender [parallel]
        en,du:
        [defObjSeen,defObjDist,defObjAng]=detectObj(def.objectDetections,1);
        settings: executionOrder=4
      state MidFielder [parallel]
        en,du:
        [midObjSeen,midObjDist,midObjAng]=detectObj(mid.objectDetections,1);
        settings: executionOrder=1
      state Striker [parallel]
        en,du:
        [stkObjSeen,stkObjDist,stkObjAng]=detectObj(stk.objectDetections,1);
        settings: executionOrder=2
        state StayStationery
          en,du:
          [stkObjSeen,stkObjDist,stkObjAng]=detectObj(stk.objectDetections,1);
          nextVel.stk = [0;0;-0.02];
        state GoToBall
          en,du:
          nextVel.stk=trackDetection(stkObjDist,stkObjAng);
        (default) -> StayStationery
        StayStationery -> GoToBall : [stkObjSeen&&stkObjDist<2.5&&stkObjAng<pi/8]
    (default) -> (junction 172)
    (junction 225) -> Attack : [awayTeam.possessingTeam==2]
    (junction 226) -> (junction 225)
    (junction 172) -> Attack [order 1] : [awayTeam.possessingTeam==2]
    (junction 172) -> (junction 173) [order 2]
    Attack -> Defend : [awayTeam.possessingTeam==1]
    Defend -> Attack [order 1] : [awayTeam.possessingTeam==2]
    (junction 173) -> Defend [order 1] : [awayTeam.possessingTeam==1]
    (junction 173) -> (junction 191) [order 2]
    CaptureBall -> Defend [order 1] : [awayTeam.possessingTeam==2]
    Defend -> CaptureBall [order 2] : [awayTeam.possessingTeam==0]
    CaptureBall -> (junction 226) [order 2]
    (junction 191) -> CaptureBall
  state [vel,done] = goToPose(goal,position) [function]
    note: Tracks a position. Once reached, the robot will turn in place until a reference angle is met.
    (default) -> (junction 9) : {
        | vel = [0;0;0];
        | [goalDist,goalAng] = calcBearing(goal(1:2),position);
        | trackAng = angdiff(position(3),goal(3));
        | }
    (junction 9) -> (junction 10) [order 1] : % Track the position if outside the distance threshold
        | [goalDist > distThresh]
    (junction 9) -> (junction 11) [order 2] : % Else, turn in place until the angular reference is met
    (junction 10) -> (junction 18) : {vel = trackDetection(goalDist,goalAng);}
    (junction 11) -> (junction 12) [order 1] : [trackAng > angThresh]
    (junction 11) -> (junction 13) [order 2]
    (junction 12) -> (junction 17) : {vel(3) = 1;}
    (junction 13) -> (junction 14) [order 1] : [trackAng < -angThresh]
    (junction 13) -> (junction 15) [order 2]
    (junction 14) -> (junction 16) : {vel(3) = -1;}
    (junction 16) -> (junction 15)
    (junction 17) -> (junction 16)
    (junction 18) -> (junction 17)
    (junction 15) -> (junction 19) : {done = (goalDist <= distThresh) && (abs(trackAng) <= angThresh);}
  state [dist,ang] = calcBearing(goal,position) [function]
    (default) -> (junction 39) : % Calculate distance and angle to location
        | {
        | err = goal(1:2) - [position(1) position(2)];
        | dist = norm(err);
        | ang = angdiff(position(3),atan2(err(2),err(1)));
        | }
  state [vel,done] = turnToPoint(goal) [function]
    note: Tracks a position. Once reached, the robot will turn in place until a reference angle is met.
    (default) -> (junction 82) : % Turn in place until the angular reference is met
        | {
        | done = false;
        | vel = [0;0;0];
        | [goalDist,goalAng] = calcBearing(goal(1:2));
        | }
    (junction 82) -> (junction 83) [order 1] : [goalAng > angThresh]
    (junction 82) -> (junction 84) [order 2]
    (junction 83) -> (junction 88) : {vel(3) = 1;}
    (junction 84) -> (junction 85) [order 1] : [goalAng < -angThresh]
    (junction 84) -> (junction 86) [order 2] : {done = true;}
    (junction 85) -> (junction 87) : {vel(3) = -1;}
    (junction 87) -> (junction 86)
    (junction 88) -> (junction 87)
  state vel = trackDetection(dist,ang) [function]
    note: Uses range and bearing to track an object
    (default) -> (junction 46) : {
        | vel = [0;0;0];
        | }
    (junction 46) -> (junction 45) [order 1] : % Turn in place
        | % if no detection
        | [dist < 0]
    (junction 45) -> (junction 55) : {vel(3) = 1;}
    (junction 46) -> (junction 47) [order 2]
    (junction 47) -> (junction 48) [order 1] : % Forward speed
        | [dist > distThresh]
    (junction 48) -> (junction 50) : {vel(1) = maxSpeed;}
    (junction 47) -> (junction 49) [order 2]
    (junction 50) -> (junction 49)
    (junction 49) -> (junction 51)
    (junction 51) -> (junction 52) [order 1] : % Turning speed
        | [ang > angThresh]
    (junction 52) -> (junction 58) : {vel(3) = maxTurnSpeed;}
    (junction 51) -> (junction 53) [order 2]
    (junction 53) -> (junction 54) [order 1] : [ang < -angThresh]
    (junction 53) -> (junction 56) [order 2]
    (junction 54) -> (junction 57) : {vel(3) = -1;}
    (junction 55) -> (junction 56)
    (junction 57) -> (junction 56)
    (junction 58) -> (junction 57)
  data: vel function_output; done function_output; goal function_input; position function_input; goal function_input; dist function_output; ang function_output; position function_input; goal function_input; vel function_output; done function_output; dist function_input; ang function_input; vel function_output; detections function_input; obj function_input; objSeen function_output; objRange function_output; objAngle function_output; awayTeam input Bus: gameSituationBus; gk input Bus: PlayerStateBus; def input Bus: PlayerStateBus; defObjSeen local boolean =false; defObjAng local =0; defObjDist local =-1; mid input Bus: PlayerStateBus; midObjSeen local boolean =false; midObjDist local =-1; midObjAng local =0; stk input Bus: PlayerStateBus; stkObjAng local =0; stkObjDist local =-1; stkObjSeen local boolean =false; toBall output; nextVel output Bus: nextVel; gkObjAng local =0; gkObjDist local =-1; gkObjSeen local boolean =false; maxSpeed parameter; maxTurnSpeed parameter; distThresh parameter; angThresh parameter; playerIdx parameter; stkPos local size=[3]
  function [objSeen, objRange,objAngle] = detectObj(detections,obj):
    | function [objSeen, objRange,objAngle] = detectObj(detections,obj)
    | % Accepts a set of object detections and searches for a ball
    | %
    | % Copyright 2019 The MathWorks, Inc.
    | objSeen = 0;
    | objRange = -1;
    | objAngle =  0;
    | 
    | objSeen = ~isempty(find(detections(:,3)==obj,1));
    | 
    | for idx = 1:size(detections,1)
    |     if detections(idx,3) == obj
    |         objRange = detections(idx,1);
    |         objAngle = detections(idx,2);
    |     end
    | end
    | 
    | end

== matlab function TDPBehaviourSim2/Game Visualiser/Plot Soccer Field ==
function plotSoccerField
% Plots the soccer field once the figure window for the environment has
% been initialized

coder.extrinsic('evalin');
persistent hasPlotted
if isempty(hasPlotted)
    evalin('base','plotSoccerField');
    hasPlotted = true;
end

== matlab function TDPBehaviourSim2/Game Visualiser/Subsystem/Object Matrix Creator ==
  data: BallPos input; objectPositions output; goalPosts input
function objectPositions = SetPositions(BallPos,goalPosts)

objectPositions =[BallPos(1) BallPos(2) 1;goalPosts];

== stateflow chart TDPBehaviourSim2/GameState ==
  state BallDynamics [parallel]
    en:
    setBallState(fieldCenter,0,0);
    settings: executionOrder=2
    state InBounds
      en:
      randNum = randn(1,2);
      du:
      gamestate.state = getGameState;
      state BallFree
      state BallHeld
        en,du:
        ballPose = [robo_pos(3*holder_idx-2) robo_pos(3*holder_idx-1)] + ...
        (playerRadius+ballThresh)*[cos(robo_pos(3*holder_idx)) sin(robo_pos(3*holder_idx))];
      (default) -> BallFree
      BallHeld -> BallFree : after(1,sec)[ballKicked==1]{setBallState(ballPose,ballVel + ballVelNoise,robo_pos(3*holder_idx))}
      BallFree -> BallHeld : [gamestate.possession(1)~=0]
    state OutOfBounds
      en,du:
      gamestate.state = getGameState;
      setBallState(ballPose,0,0);
      if lastPossession == 1
      end
    state CornerOrGOakKick
      en,du:
      gamestate.state = getGameState;
    state GoalScored
      en,du:
      gamestate.state = getGameState;
    (default) -> InBounds
    OutOfBounds -> InBounds : [gamestate.state==gameSituation(1)]
    InBounds -> OutOfBounds [order 1] : [gamestate.state == gameSituation(2)]
    GoalScored -> InBounds : [gamestate.state==gameSituation(1)]
    InBounds -> GoalScored [order 2] : [gamestate.state==gameSituation(3)]
    CornerOrGOakKick -> InBounds : [gamestate.state==gameSituation(1)]
    InBounds -> CornerOrGOakKick [order 3] : [gamestate.state==gameSituation(4)]
  state TimeSetter [parallel]
    en,du:
    settings: executionOrder=3
    state EarlyGame
      en,du:
      time=elapsed(sec);
      gamestate.time=gameTime(1);
    state MidGame
      en,du:
      time=elapsed(sec);
      gamestate.time=gameTime(2);
    state LateGame
      en,du:
      time=elapsed(sec);
      gamestate.time=gameTime(3)
    state GameOver
      en:
      done = 1;
    (default) -> EarlyGame
    EarlyGame -> MidGame : [time==400]
    MidGame -> LateGame : [time==800]
    LateGame -> GameOver : [time==1200]
  state state = getGameState [function]
    note: Returns the game state depending on the position of the ball on the field
    (default) -> (junction 52)
    (junction 52) -> (junction 53) [order 1] : [ballPose(1) <= fieldLimitsX(1) || ballPose(1) >= fieldLimitsX(2) || ...
        |  ballPose(2) <= fieldLimitsY(1) || ballPose(2) >= fieldLimitsY(2)]
    (junction 52) -> (junction 56) [order 2] : {state = gameSituation.InPlay;}
    (junction 53) -> (junction 54)
    (junction 54) -> (junction 55) [order 1] : [ballPose(2)<=goalPosts(1,2) && ...
        | ballPose(2) >= goalPosts(2,2)]
    (junction 54) -> (junction 57) [order 2] : {state = gameSituation.OutOfPlay;}
    (junction 55) -> (junction 58) : {state = gameSituation.GoalScored;}
    (junction 57) -> (junction 56)
    (junction 58) -> (junction 57)
  state setBallState(pos,vel,theta) [function]
  state DeterminePossession [parallel]
    en,du:
    gamestate.possession = [holded,holder_idx];
    if gamestate.possession(2)>0 &&gamestate.possession(2)<=4
    gamestate.possessingTeam = 1;
    lastPossession = 1;
    elseif gamestate.possession(2)>=5
    gamestate.possessingTeam = 2;
    lastPossession = 2;
    else
    gamestate.possessingTeam = 0;
    end
    settings: executionOrder=1
  data: sf_internal_action_state_placeholder_data local double size=1 =0; state function_output; pos function_input double size=[1 2]; vel function_input double size=1; theta function_input double size=1; ballPose output =fieldCenter; attackerKickSpeed parameter; ballThresh parameter; ballDist local; playerRadius parameter double; fieldLimitsX parameter; fieldLimitsY parameter; goalPosts parameter; fieldCenter parameter; robo_pos input; gamestate output Bus: gameSituationBus; ballVel local =0.5; ballVelNoise parameter; ballAngleNoise parameter; randNum local =[0 0]; ballKicked local =0; time local; done output =0; lastPossession local =0; holded input; holder_idx input

== matlab function TDPBehaviourSim2/MATLAB Function ==
  data: home input; holded output; away input; indexholder output
function [holded,indexholder]=findholder(home,away)
holded=false;
holdingTeam= 0;
indexholder=0;
awayHolds=0;
homeHolds=0;
determineholder=0;
%% This function returns if ball is holded or not and the player's index if holded
homeindexholder = find(home(:,1) ~= 0 & home(:,2) < 0.3  & home(:,2) > 0  & home(:,3) > -pi/4 & home(:,3) < pi/4);
awayindexholder = find(away(:,1) ~= 0 & away(:,2) < 0.3 & away(:,2) > 0 & away(:,3) >-pi/4  & away(:,3) < pi/4);
awayHolds = ~isempty(awayindexholder);
homeHolds = ~isempty(homeindexholder);

if awayHolds || homeHolds
    holded = true;
    if homeHolds && ~awayHolds
        if size(homeindexholder,1)== 1
            indexholder = homeindexholder(1);
        else
            indexholder = homeindexholder(randi([1,size(homeindexholder,1)]));            
        end
    elseif awayHolds && ~homeHolds
        if size(homeindexholder,1)>1
            indexholder = awayindexholder(randi([1,size(awayindexholder,1)])) + 4;
        else
            indexholder = awayindexholder(1);
        end
    elseif  homeHolds && awayHolds
        determineholder = [homeindexholder;awayindexholder+4];
        indexholder = determineholder(randi([1,size(determineholder,1)]));
    end
    
end
end
